simulink model "Three_Ph_inverter"  (R2019a)
settings: Solver=VariableStepAuto  StartTime=0.0  StopTime=1.0  RelTol=1e-3
libraries: powerlib x15
settings Model: Creator=Amanna  LastModifiedBy=Amanna

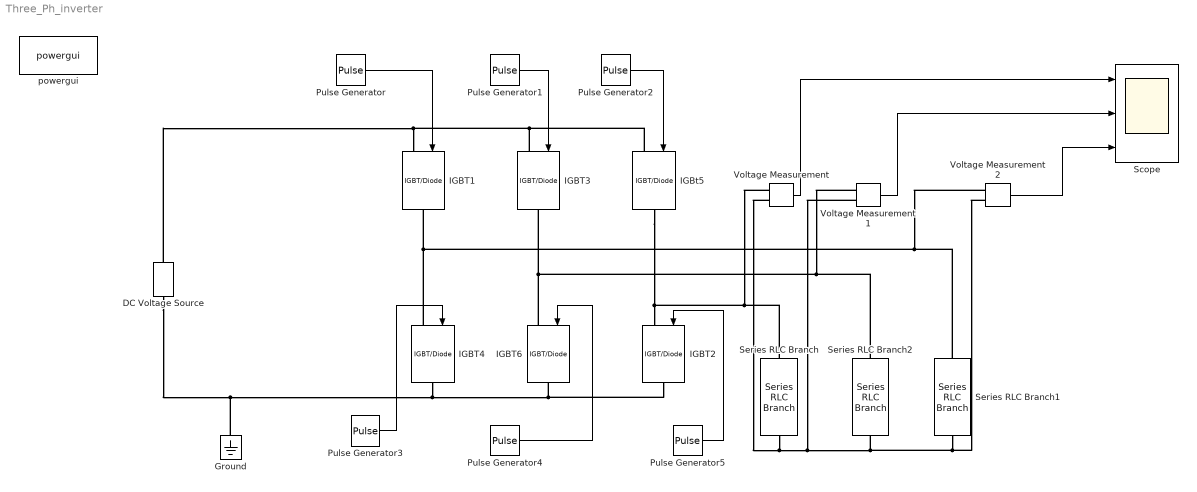
== system Three_Ph_inverter ==
  DC Voltage Source : powerlib/Electrical Sources/DC Voltage Source  Amplitude=100  Measurements=None
      settings: SourceProductName=Simscape Electrical
  Ground : powerlib/Elements/Ground  LConnTagsString=a
      settings: SourceProductName=Simscape Electrical
  IGBT{1..4,6} (5 alike) : powerlib/Power Electronics/IGBT//Diode  Ron=1e-3  Rs=1e5  Cs=inf  Measurements=off
      settings: SourceProductName=Simscape Electrical
  IGBt5 : powerlib/Power Electronics/IGBT//Diode  Ron=1e-3  Rs=1e5  Cs=inf  Measurements=off
      settings: SourceProductName=Simscape Electrical
  Pulse Generator : DiscretePulseGenerator  PulseType=Time based  Period=2e-3  PulseWidth=50
  Pulse Generator1 : DiscretePulseGenerator  PulseType=Time based  Period=2e-3  PulseWidth=50  PhaseDelay=2e-3*(1/3)
  Pulse Generator2 : DiscretePulseGenerator  PulseType=Time based  Period=2e-3  PulseWidth=50  PhaseDelay=2e-3*(2/3)
  Pulse Generator3 : DiscretePulseGenerator  PulseType=Time based  Period=2e-3  PulseWidth=50  PhaseDelay=2e-3*(1/2)
  Pulse Generator4 : DiscretePulseGenerator  PulseType=Time based  Period=2e-3  PulseWidth=50  PhaseDelay=2e-3*(5/6)
  Pulse Generator5 : DiscretePulseGenerator  PulseType=Time based  Period=2e-3  PulseWidth=50  PhaseDelay=2e-3*(1/6)
  Scope : Scope  NumInputPorts=3
  Series RLC Branch : powerlib/Elements/Series RLC Branch  LConnTagsString=__new0  RConnTagsString=__new0  BranchType=R  Resistance=10  Inductance=1e-3  SetiL0=off  InitialCurrent=0  Capacitance=1e-6  Setx0=off  InitialVoltage=0  Measurements=None
      settings: SourceProductName=Simscape Electrical
  Series RLC Branch1 : powerlib/Elements/Series RLC Branch  LConnTagsString=__new0  RConnTagsString=__new0  BranchType=R  Resistance=10  Inductance=1e-3  SetiL0=off  InitialCurrent=0  Capacitance=1e-6  Setx0=off  InitialVoltage=0  Measurements=None
      settings: SourceProductName=Simscape Electrical
  Series RLC Branch2 : powerlib/Elements/Series RLC Branch  LConnTagsString=__new0  RConnTagsString=__new0  BranchType=R  Resistance=10  Inductance=1e-3  SetiL0=off  InitialCurrent=0  Capacitance=1e-6  Setx0=off  InitialVoltage=0  Measurements=None
      settings: SourceProductName=Simscape Electrical
  Voltage Measurement : powerlib/Measurements/Voltage Measurement  PhasorSimulation=off  OutputType=Complex  PSBequivalent=0
      settings: SourceProductName=Simscape Electrical
  Voltage Measurement1 : powerlib/Measurements/Voltage Measurement  PhasorSimulation=off  OutputType=Complex  PSBequivalent=0
      settings: SourceProductName=Simscape Electrical
  Voltage Measurement2 : powerlib/Measurements/Voltage Measurement  PhasorSimulation=off  OutputType=Complex  PSBequivalent=0
      settings: SourceProductName=Simscape Electrical
  powergui : powerlib/powergui  Priority=1  SimulationMode=Continuous  SampleTime=50e-6  frequency=60  Iterations=50  frequencyindice=0  Pbase=100e6  ErrMax=1e-4  UnitsV=kV  UnitsW=MW  buscounter=0  FunctionMessages=off  echomessages=off  EnableUseOfTLC=off  CurrentSourceSwitches=off  DisableSnubberDevices=off  DisableRonSwitches=off  DisableVfSwitches=off  DisplayEquations=off  AutomaticDiscreteSolvers=off  SolverType=Tustin/Backward Euler (TBE)  Interpol=off  ExternalGateDelay=off  methode=off  Ts=100  x0status=blocks  SPID=on  SwTol=0  HookPort=off  NonlinearTolerance=0  nMaxIteration=15  ContinueOnMaxIteration=off  RestoreLinks=warning  ResistiveCurrentMeasurement=off  Frange=[0:2:500]  Ylog=off  Xlog=on  ShowGrid=off  save=off  variable=ZData  structure=0  ZoomFFT=off  StartTime=0.0  cycles=1  DisplayStyle=1  fundamental=60  FreqAxis=off  MaxFrequency=1000  frequencyindicesteady=1  RmsSteady=1  display=off
      settings: SourceProductName=Simscape Electrical
  wires:
  Pulse Generator/1 -> IGBT1/1
  Pulse Generator1/1 -> IGBT3/1
  Pulse Generator2/1 -> IGBt5/1
  Pulse Generator3/1 -> IGBT4/1
  Pulse Generator4/1 -> IGBT6/1
  Pulse Generator5/1 -> IGBT2/1
  Voltage Measurement2/1 -> Scope/3
  Voltage Measurement1/1 -> Scope/2
  Voltage Measurement/1 -> Scope/1
  connections:
  IGBT3/LConn1 -- DC Voltage Source/RConn1 -- IGBT1/LConn1 -- IGBt5/LConn1
  IGBT4/RConn1 -- Ground/LConn1 -- DC Voltage Source/LConn1 -- IGBT2/RConn1 -- IGBT6/RConn1
  IGBT4/LConn1 -- Voltage Measurement2/LConn1 -- Series RLC Branch1/LConn1 -- IGBT1/RConn1
  IGBT6/LConn1 -- Voltage Measurement1/LConn1 -- Series RLC Branch2/LConn1 -- IGBT3/RConn1
  IGBt5/RConn1 -- Voltage Measurement/LConn1 -- Series RLC Branch/LConn1 -- IGBT2/LConn1
  Series RLC Branch/RConn1 -- Voltage Measurement/LConn2 -- Series RLC Branch1/RConn1 -- Voltage Measurement2/LConn2 -- Series RLC Branch2/RConn1 -- Voltage Measurement1/LConn2
